simulink model "my_turn_pp"  (R2020a)
settings: Solver=FixedStepAuto  StartTime=0.0  StopTime=30  FixedStep=.01  RelTol=1e-3
undefined symbols (not defined in the file or in its folder): angdiff
libraries: simulink x2
settings Model: Creator=Jamie  LastModifiedBy=Jamie

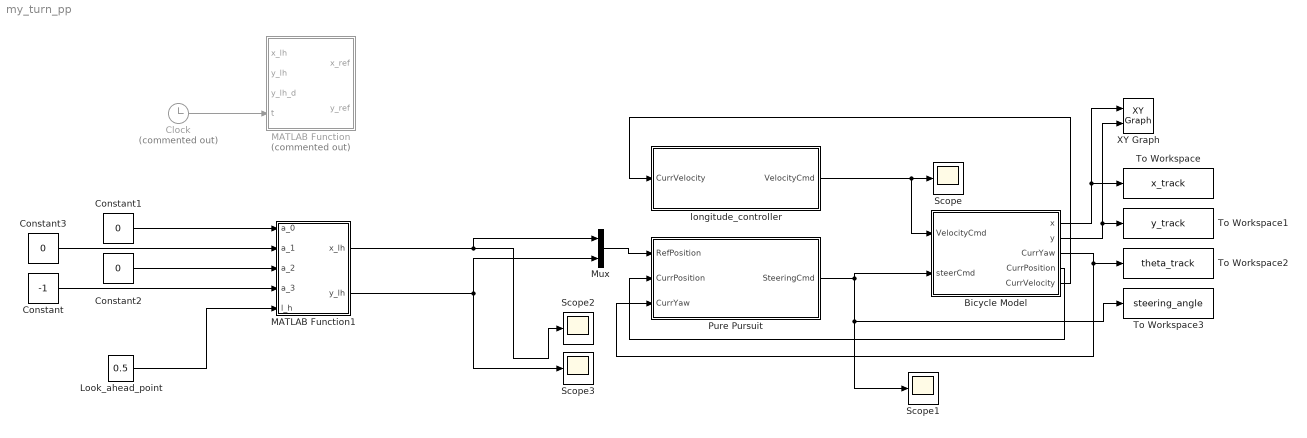
== system my_turn_pp ==
  Bicycle Model : Subsystem
  Clock : Clock  Commented=on
  Constant : Constant  Value=-1
  Constant1 : Constant  Value=0
  Constant2 : Constant  Value=0
  Constant3 : Constant  Value=0
  Look_ahead_point : Constant  Value=0.5
  MATLAB Function : MATLAB Function  Commented=on  TreatAsAtomicUnit=on
  MATLAB Function1 : MATLAB Function  TreatAsAtomicUnit=on
  Mux : Mux  Inputs=2
  Pure Pursuit : Subsystem
  Scope{,1..3} (4 alike) : Scope
  To Workspace : ToWorkspace  VariableName=x_track  SampleTime=-1
      settings: Save2DSignal=2-D array (concatenate along first dimension)
  To Workspace1 : ToWorkspace  VariableName=y_track  SampleTime=-1
      settings: Save2DSignal=2-D array (concatenate along first dimension)
  To Workspace2 : ToWorkspace  VariableName=theta_track  SampleTime=-1
      settings: Save2DSignal=2-D array (concatenate along first dimension)
  To Workspace3 : ToWorkspace  VariableName=steering_angle  SampleTime=-1
      settings: Save2DSignal=2-D array (concatenate along first dimension)
  XY Graph : simulink/Sinks/XY Graph  xmin=-2.5  xmax=2.5  ymin=-2.5  ymax=2.5  st=-1
  longitude_controller : Subsystem
  wires:
  Bicycle Model/4(CurrPosition) -> Pure Pursuit/2(CurrPosition)
  Pure Pursuit/1(SteeringCmd) -> Bicycle Model/2(steerCmd), Scope1/1, To Workspace3/1
  Bicycle Model/3(CurrYaw) -> To Workspace2/1, Pure Pursuit/3(CurrYaw)
  Bicycle Model/1(x) -> XY Graph/1, To Workspace/1
  Bicycle Model/2(y) -> XY Graph/2, To Workspace1/1
  Bicycle Model/5(CurrVelocity) -> longitude_controller/1(CurrVelocity)
  longitude_controller/1(VelocityCmd) -> Scope/1, Bicycle Model/1(VelocityCmd)
  Look_ahead_point/1 -> MATLAB Function1/5(l_h)
  Constant/1 -> MATLAB Function1/4(a_3)
  Constant2/1 -> MATLAB Function1/3(a_2)
  Constant1/1 -> MATLAB Function1/1(a_0)
  Constant3/1 -> MATLAB Function1/2(a_1)
  Mux/1 -> Pure Pursuit/1(RefPosition)
  Clock/1 -> MATLAB Function/4(t)
  MATLAB Function1/1(x_lh) -> Scope2/1, Mux/1
  MATLAB Function1/2(y_lh) -> Scope3/1, Mux/2

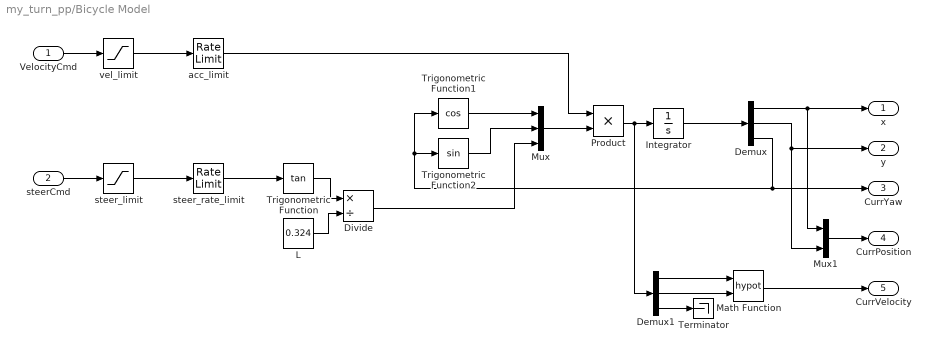
== system my_turn_pp/Bicycle Model ==
  VelocityCmd : Inport
  steerCmd : Inport  Port=2
  Demux : Demux  Outputs=3
  Demux1 : Demux  Outputs=3
  Divide : Product  Inputs=*/
  Integrator : Integrator  InitialCondition=[0, 0, pi/2]
  L : Constant  Value=0.324
  Math Function : Math  Operator=hypot  SaturateOnIntegerOverflow=on
  Mux : Mux  Inputs=3
  Mux1 : Mux  Inputs=2
  Product : Product
  Terminator : Terminator
  Trigonometric Function : Trigonometry  Operator=tan
  Trigonometric Function1 : Trigonometry  Operator=cos
  Trigonometric Function2 : Trigonometry
  acc_limit : RateLimiter  SampleTimeMode=inherited
  steer_limit : Saturate
  steer_rate_limit : RateLimiter  RisingSlewLimit=3  FallingSlewLimit=-3  SampleTimeMode=inherited
  vel_limit : Saturate  UpperLimit=3  LowerLimit=-3
  x : Outport
  y : Outport  Port=2
  CurrYaw : Outport  Port=3
  CurrPosition : Outport  Port=4
  CurrVelocity : Outport  Port=5
  wires:
  steerCmd/1 -> steer_limit/1
  VelocityCmd/1 -> vel_limit/1
  vel_limit/1 -> acc_limit/1
  steer_limit/1 -> steer_rate_limit/1
  steer_rate_limit/1 -> Trigonometric Function/1
  Trigonometric Function/1 -> Divide/1
  L/1 -> Divide/2
  acc_limit/1 -> Product/1
  Trigonometric Function1/1 -> Mux/1
  Trigonometric Function2/1 -> Mux/2
  Mux/1 -> Product/2
  Product/1 -> Demux1/1, Integrator/1
  Divide/1 -> Mux/3
  Integrator/1 -> Demux/1
  Demux/1 -> Mux1/1, x/1
  Demux/2 -> Mux1/2, y/1
  Demux/3 -> Trigonometric Function1/1, Trigonometric Function2/1, CurrYaw/1
  Mux1/1 -> CurrPosition/1
  Demux1/1 -> Math Function/1
  Demux1/2 -> Math Function/2
  Demux1/3 -> Terminator/1
  Math Function/1 -> CurrVelocity/1

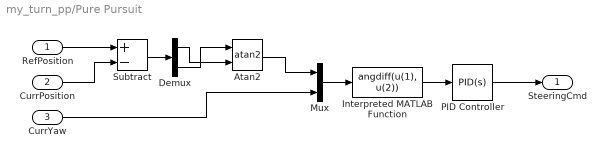
== system my_turn_pp/Pure Pursuit ==
  RefPosition : Inport
  CurrPosition : Inport  Port=2
  CurrYaw : Inport  Port=3
  Atan2 : Trigonometry  Operator=atan2
  Demux : Demux  Outputs=2
  Interpreted MATLAB Function : MATLABFcn  MATLABFcn=angdiff(u(1), u(2))
  Mux : Mux  Inputs=2
  PID Controller : simulink/Continuous/PID Controller  Controller=PID  Form=Parallel  TimeDomain=Continuous-time  UseExternalTs=off  SampleTime=-1  IntegratorMethod=Forward Euler  FilterMethod=Forward Euler  ControllerParametersSource=internal  P=-0.5  I=0  D=0  UseFilter=on  N=100  TunerSelectOption=Transfer Function Based (PID Tuner App)  InitialConditionSource=internal  InitialConditionForIntegrator=0  InitialConditionForFilter=0  DifferentiatorICPrevScaledInput=0  ExternalReset=none  TrackingMode=off  Kt=1  LimitOutput=off  UpperSaturationLimit=inf  LowerSaturationLimit=-inf  LinearizeAsGain=on  AntiWindupMode=none  Kb=1  POutMin=[]  POutMax=[]  IOutMin=[]  IOutMax=[]  DOutMin=[]  DOutMax=[]  NOutMin=[]  NOutMax=[]  SumOutMin=[]  SumOutMax=[]  SaturationOutMin=[]  SaturationOutMax=[]  PParamMin=[]  PParamMax=[]  IParamMin=[]  IParamMax=[]  DParamMin=[]  DParamMax=[]  NParamMin=[]  NParamMax=[]  KbParamMin=[]  KbParamMax=[]  KtParamMin=[]  KtParamMax=[]  KbOutMin=[]  KbOutMax=[]  KtOutMin=[]  KtOutMax=[]  IntegratorOutMin=[]  IntegratorOutMax=[]  FilterOutMin=[]  FilterOutMax=[]  SumI1OutMin=[]  SumI1OutMax=[]  SumI2OutMin=[]  SumI2OutMax=[]  SumI3OutMin=[]  SumI3OutMax=[]  SumI4OutMin=[]  SumI4OutMax=[]  SumDOutMin=[]  SumDOutMax=[]  DifferentiatorOutMin=[]  DifferentiatorOutMax=[]  FilterDiffOutCoefMin=[]  FilterDiffOutCoefMax=[]  ReciprocalOutMin=[]  ReciprocalOutMax=[]  SumDenOutMin=[]  SumDenOutMax=[]  SumNumOutMin=[]  SumNumOutMax=[]  DivideOutMin=[]  DivideOutMax=[]  UdiffTsProdOutMin=[]  UdiffTsProdOutMax=[]  NTsProdOutMin=[]  NTsProdOutMax=[]  UintegralTsProdOutMin=[]  UintegralTsProdOutMax=[]  UngainTsProdOutMin=[]  UngainTsProdOutMax=[]  IntegratorContinuousStateAttributes=''  IntegratorStateMustResolveToSignalObject=off  IntegratorRTWStateStorageClass=Auto  FilterContinuousStateAttributes=''  FilterStateMustResolveToSignalObject=off  FilterRTWStateStorageClass=Auto  ParallelPVariant=InternalParameters  IdealPVariant=Disabled  IVariant=InternalParameters  DVariant=InternalParameters  IntegratorVariant=Continuous  SatVariant=Disabled  AWVariant=Passthrough  PCopyVariant=Disabled  TRVariant=Disabled  FdbkBlocksVariant=Forward  IdealPFdbkVariant=Disabled  SatFdbkVariant=Disabled  DerivativeFilterVariant=ContFilter  NVariant=InternalParameters  NCopyVariant=Disabled  FilterICVariant=InternalICsFilter  IntegratorICVariant=InternalICs  ExternalResetVariant=Disabled  TRSumVariant=Passthrough  SumFdbkVariant=Disabled  SumVariant=Sum_PID  TsampFilterVariant=InternalTs  TsampNgainVariant=Passthrough  TsampIntegralVariant=Passthrough
  Subtract : Sum  Inputs=+-
  SteeringCmd : Outport
  wires:
  RefPosition/1 -> Subtract/1
  CurrPosition/1 -> Subtract/2
  Subtract/1 -> Demux/1
  Demux/2 -> Atan2/1
  Demux/1 -> Atan2/2
  Mux/1 -> Interpreted MATLAB Function/1
  Atan2/1 -> Mux/1
  CurrYaw/1 -> Mux/2
  Interpreted MATLAB Function/1 -> PID Controller/1
  PID Controller/1 -> SteeringCmd/1

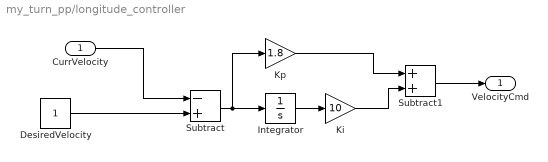
== system my_turn_pp/longitude_controller ==
  CurrVelocity : Inport
  DesiredVelocity : Constant
  Integrator : Integrator
  Ki : Gain  Gain=10
  Kp : Gain  Gain=1.8
  Subtract : Sum  Inputs=-+
  Subtract1 : Sum
  VelocityCmd : Outport
  wires:
  Subtract1/1 -> VelocityCmd/1
  DesiredVelocity/1 -> Subtract/2
  Ki/1 -> Subtract1/2
  Subtract/1 -> Integrator/1, Kp/1
  Integrator/1 -> Ki/1
  Kp/1 -> Subtract1/1
  CurrVelocity/1 -> Subtract/1

== matlab function my_turn_pp/MATLAB Function1 ==
  data: x_lh output; y_lh output; a_0 input; a_1 input; a_2 input; a_3 input; l_h input
function [x_lh,y_lh] = fcn(a_0, a_1, a_2, a_3, l_h)
i = 0;
    
while(1)
    x_t = l_h - i;
    y_t = a_3*x_t^3 + a_2*x_t^2 + a_1*x_t + a_0;
    
    d_t = sqrt(x_t^2 + y_t^2);
    if(x_t <= 0.01)
        x_lh = l_h;
        y_lh = 0;
%         y_lh_d = 0
        break
    else
        if(abs(d_t - l_h) <= 0.01)
            x_lh = x_t;
            y_lh = y_t;
%             y_lh_d = 3*a_3*x_t^2 + 2*a_2*x_t + a_1;
            break;  
        else
            i = i + 0.01;
        end
    end
  
end

== matlab function my_turn_pp/MATLAB Function ==
  data: x_lh input; x_ref output; y_lh input; y_lh_d input; y_ref output; t input
function [x_ref, y_ref] = fcn(x_lh, y_lh, y_lh_d, t)

t = 0.01*mod(1000*t, 10);
x_ref = (3*t^2 - 2*t^3)*x_lh + (-2*t^2 + t^3 + t) + (-t^2 + t^3)*(1/(1 + y_lh_d^2));
y_ref = (3*t^2 - 2*t^3)*y_lh + (-t^2 + t^3)*(y_lh_d/(1 + y_lh_d^2));

end
